simulink model "RaspPiPilot"  (R2014a)
settings: Solver=FixedStepDiscrete  SolverMode=SingleTasking  StartTime=0.0  StopTime=inf  FixedStep=0.2  RelTol=1e-3
PreLoadFcn:
  | load JoystickBus
undefined symbols (not defined in the file or in its folder): fdesignblkfcn, gcbh
libraries: simulink x11, visionstatistics x5, visiontextngfix x2, embdlinuxlib x2
settings Model: SimulationMode=external  ExtModeTrigDuration=100  Creator=jsustare  LastModifiedBy=jsustare
settings OptimizationCC: OptimizeModelRefInitCode=on  LifeSpan=1
settings DebuggingCC: UnderspecifiedInitializationDetection=Classic  SolverPrmCheckMsg=none
settings HardwareCC: ProdLargestAtomicInteger=Long  ProdLargestAtomicFloat=Double  ProdEndianess=LittleEndian  ProdHWDeviceType=ARM Compatible->ARM Cortex
settings RTWCC: SystemTargetFile=realtime.tlc  GenerateMakefile=off  TemplateMakefile=realtime.tmf  Description=Run on Target Hardware  RTWVerbose=off  ProcessScript=realtime_make_rtw_hook  CustomInclude=include include/common  CustomSource=SerialPort.c mavlink.c
settings RTWCC: CustomHeaderCode=|
  | #include <mavlink.h>
  | #include <common.h>
settings STFCustomTargetCC: TargetLibSuffix=.a  GenerateSampleERTMain=on  ConcurrentExecutionCompliant=off  GeneratePreprocessorConditionals=Use local settings  ERTCustomFileBanners=on  SupportNonInlinedSFcns=off  SupportVariableSizeSignals=on  MATLABClassNameForMDSCustomization=Simulink.SoftwareTarget.ERTCustomization  GRTInterface=off  SystemTargetFile=realtime.tlc
settings ERTTargetCC: CombineOutputUpdateFcns=off  SupportContinuousTime=on  SupportVariableSizeSignals=on  ExtMode=on  ExtModeMexArgs='169.254.0.31' 0 17725 30  ERTSrcFileBannerTemplate=realtime_code_template.cgt  ERTHdrFileBannerTemplate=realtime_code_template.cgt  ERTDataSrcFileTemplate=realtime_code_template.cgt  ERTDataHdrFileTemplate=realtime_code_template.cgt  ERTCustomFileTemplate=realtime_file_process.tlc

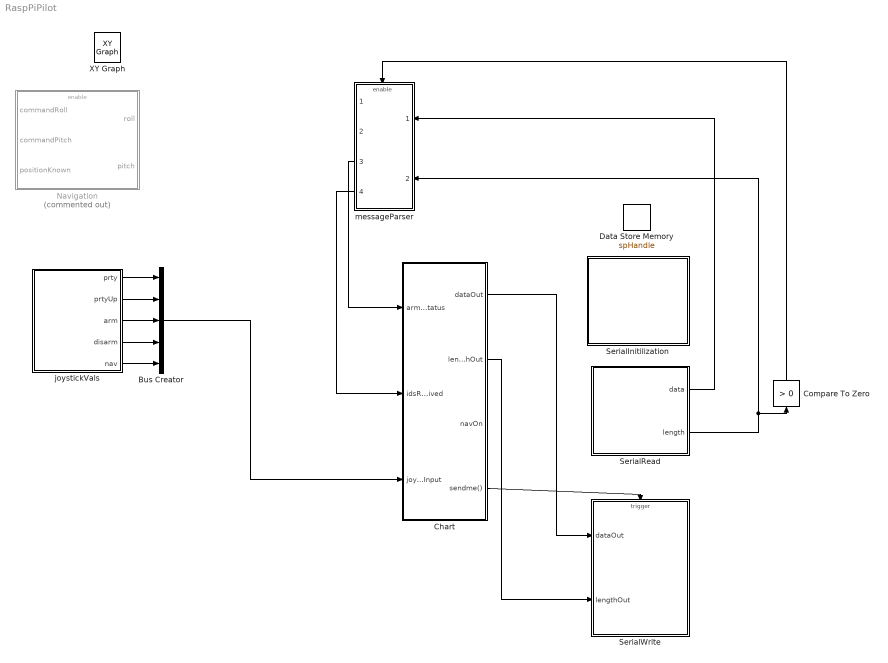
== system RaspPiPilot ==
  Bus Creator : BusCreator  Inputs=5  OutDataTypeStr=Bus: JoystickBus
  Chart : Stateflow chart  TreatAsAtomicUnit=on
  Compare To Zero : simulink/Logic and Bit Operations/Compare To Zero  relop=>  OutDataTypeStr=boolean
  Data Store Memory : DataStoreMemory  DataStoreName=spHandle  ReadBeforeWriteMsg=warning  WriteAfterWriteMsg=warning  WriteAfterReadMsg=warning  InitialValue=-1  OutDataTypeStr=int32
  Navigation : Subsystem  Commented=on
  SerialInitilization : MATLAB Function  TreatAsAtomicUnit=on
  SerialRead : MATLAB Function  TreatAsAtomicUnit=on
  SerialWrite : MATLAB Function  TreatAsAtomicUnit=on
  joystickVals : Subsystem
  messageParser : Subsystem
  XY Graph : simulink/Sinks/XY Graph  IOType=viewer  xmin=-1  xmax=1  ymin=-1  ymax=1  st=-1
  wires:
  Compare To Zero/1 -> messageParser/Enable
  Chart/1(dataOut) -> SerialWrite/1(dataOut)
  Chart/2(lengthOut) -> SerialWrite/2(lengthOut)
  Chart/4(sendme()) -> SerialWrite/Trigger
  SerialRead/2(length) -> messageParser/2(lengthRead), Compare To Zero/1
  SerialRead/1(data) -> messageParser/1("dataRead ")
  messageParser/3(armStatus) -> Chart/1(armStatus)
  messageParser/4(bussyBus) -> Chart/2(idsReceived)
  joystickVals/4(disarm) -> Bus Creator/4
  joystickVals/1(prty) -> Bus Creator/1
  joystickVals/3(arm) -> Bus Creator/3
  joystickVals/2(prtyUp) -> Bus Creator/2
  joystickVals/5(nav) -> Bus Creator/5
  Bus Creator/1 -> Chart/3(joystickInput)

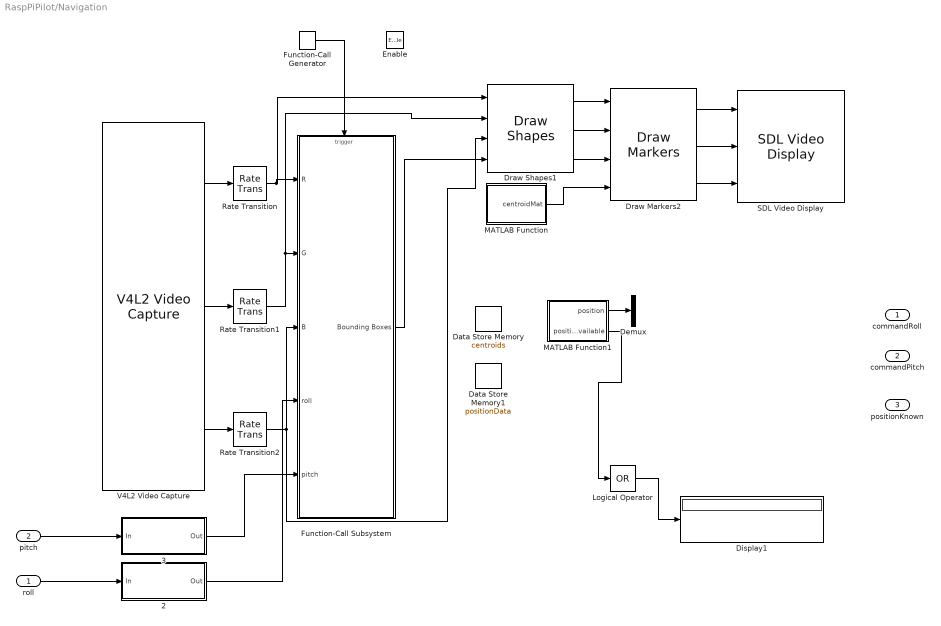
== system RaspPiPilot/Navigation ==
  roll : Inport
  pitch : Inport  Port=2
  Enable : EnablePort  PropagateVarSize=During execution
  " 2" : Subsystem  DialogController=fdesignblkfcn  InitFcn=fdesignblkfcn(gcbh, {'InitFcn'});  mask(Lowpass Filter){}
      mask help: Design a lowpass filter
      settings: CopyFcn=fdesignblkfcn(gcbh, {'CopyFcn'});
      mask Help: helpview(mapfilelocation('dsp'), 'dsplowpassfilter');
      mask Display: disp('Lowpass')
  " 3" : Subsystem  DialogController=fdesignblkfcn  InitFcn=fdesignblkfcn(gcbh, {'InitFcn'});  mask(Lowpass Filter){}
      mask help: Design a lowpass filter
      settings: CopyFcn=fdesignblkfcn(gcbh, {'CopyFcn'});
      mask Help: helpview(mapfilelocation('dsp'), 'dsplowpassfilter');
      mask Display: disp('Lowpass')
  Data Store Memory : DataStoreMemory  DataStoreName=centroids  ReadBeforeWriteMsg=warning  WriteAfterWriteMsg=warning  WriteAfterReadMsg=warning  InitialValue=zeros(13,2,4)  OutDataTypeStr=double
  Data Store Memory1 : DataStoreMemory  DataStoreName=positionData  ReadBeforeWriteMsg=warning  WriteAfterWriteMsg=warning  WriteAfterReadMsg=warning  InitialValue=-1000*ones(4,2)  OutDataTypeStr=double
  Demux : Demux  Outputs=2
  Display1 : Display
  Draw Markers2 : visiontextngfix/Draw Markers  shape=X-mark  size=3  fill=off  fillClrSource=Specify via dialog  display=User-specified value  intensity=200  color=[255 255 255]  opacity=0.6  viewport=Entire image  antialiasing=off  inType=Obsolete  imagePorts=Separate color signals  prodOutputMode=Binary point scaling  prodOutputWordLength=32  prodOutputFracLength=14  memoryMode=Specify word length  memoryWordLength=16  memoryFracLength=15  roundingMode=Floor  overflowMode=off
  Draw Shapes1 : visiontextngfix/Draw Shapes  shape=Rectangles  fill=off  lineWidth=1  fillClrSource=Specify via dialog  display=User-specified value  intensity=200  color=[255 0 0]  opacity=0.6  viewport=Entire image  antialiasing=off  inType=Obsolete  imagePorts=Separate color signals  prodOutputMode=Binary point scaling  prodOutputWordLength=32  prodOutputFracLength=14  memoryMode=Specify word length  memoryWordLength=16  memoryFracLength=15  roundingMode=Floor  overflowMode=off
  Function-Call Generator : simulink/Ports & Subsystems/Function-Call Generator  sample_time=0.2  numberOfIterations=1
  Function-Call Subsystem : Subsystem  TreatAsAtomicUnit=on
  Logical Operator : Logic  Operator=OR  Inputs=1  AllPortsSameDT=off  OutDataTypeStr=boolean
  MATLAB Function : MATLAB Function  TreatAsAtomicUnit=on
  MATLAB Function1 : MATLAB Function  TreatAsAtomicUnit=on
  Rate Transition : RateTransition  Deterministic=off
  Rate Transition1 : RateTransition  Deterministic=off
  Rate Transition2 : RateTransition  Deterministic=off
  SDL Video Display : embdlinuxlib/SDL Video Display  pixelFormat=RGB  pixelOrder=Planar  rowMajor=on  blockPlatform=Raspberry Pi
  V4L2 Video Capture : embdlinuxlib/V4L2 Video Capture  m_devName='/dev/video0'  roi=[0, 0, 640, 480]  imSizeSelection=320x240  imSize=[640, 480]  pixelFormat=RGB  pixelOrder=Planar  sampleTime=0.2  simOutput=Colorbars  blockPlatform=Raspberry Pi
  commandRoll : Outport
  commandPitch : Outport  Port=2
  positionKnown : Outport  Port=3
  wires:
  V4L2 Video Capture/3 -> Rate Transition2/1
  V4L2 Video Capture/1 -> Rate Transition/1
  V4L2 Video Capture/2 -> Rate Transition1/1
  Function-Call Generator/1 -> Function-Call Subsystem/Trigger
  Function-Call Subsystem/1("Bounding Boxes ") -> Draw Shapes1/4
  Rate Transition/1 -> Draw Shapes1/1, Function-Call Subsystem/1(R)
  Rate Transition1/1 -> Draw Shapes1/2, Function-Call Subsystem/2(G)
  Rate Transition2/1 -> Draw Shapes1/3, Function-Call Subsystem/3(B)
  Draw Markers2/2 -> SDL Video Display/2
  Draw Markers2/3 -> SDL Video Display/3
  Draw Markers2/1 -> SDL Video Display/1
  Draw Shapes1/3 -> Draw Markers2/3
  Draw Shapes1/2 -> Draw Markers2/2
  Draw Shapes1/1 -> Draw Markers2/1
  pitch/1 -> " 3"/1(In)
  " 2"/1(Out) -> Function-Call Subsystem/4(roll)
  roll/1 -> " 2"/1(In)
  MATLAB Function/1(centroidMat) -> Draw Markers2/4
  MATLAB Function1/2(positionAvailable) -> Logical Operator/1
  Logical Operator/1 -> Display1/1
  " 3"/1(Out) -> Function-Call Subsystem/5(pitch)
  MATLAB Function1/1(position) -> Demux/1

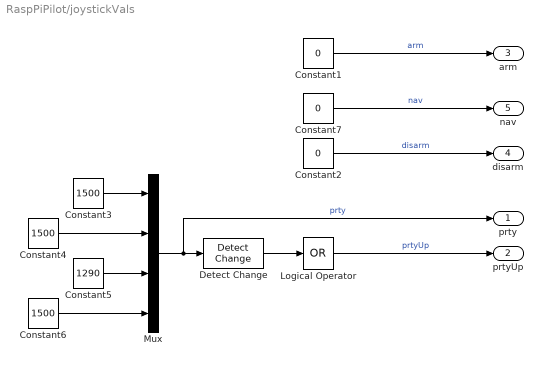
== system RaspPiPilot/joystickVals ==
  Constant1 : Constant  Value=0  OutDataTypeStr=boolean
  Constant2 : Constant  Value=0  OutDataTypeStr=boolean
  Constant3 : Constant  Value=1500
  Constant4 : Constant  Value=1500
  Constant5 : Constant  Value=1290
  Constant6 : Constant  Value=1500
  Constant7 : Constant  Value=0  OutDataTypeStr=boolean
  Detect Change : simulink/Logic and Bit Operations/Detect Change  vinit=0  InputProcessing=Inherited  OutDataTypeStr=boolean
  Logical Operator : Logic  Operator=OR  Inputs=1  AllPortsSameDT=off  OutDataTypeStr=boolean
  Mux : Mux
  prty : Outport
  prtyUp : Outport  Port=2
  arm : Outport  Port=3
  disarm : Outport  Port=4
  nav : Outport  Port=5
  wires:
  Constant3/1 -> Mux/1
  Constant4/1 -> Mux/2
  Constant5/1 -> Mux/3
  Constant6/1 -> Mux/4
  Mux/1 -> prty/1, Detect Change/1  "prty"
  Detect Change/1 -> Logical Operator/1
  Logical Operator/1 -> prtyUp/1  "prtyUp"
  Constant1/1 -> arm/1  "arm"
  Constant2/1 -> disarm/1  "disarm"
  Constant7/1 -> nav/1  "nav"

== system RaspPiPilot/messageParser ==
  "dataRead " : Inport
  lengthRead : Inport  Port=2
  Enable : EnablePort
  While Iterator Subsystem : Subsystem  TreatAsAtomicUnit=on
  rollData : Outport
  pitchData : Outport  Port=2
  armStatus : Outport  Port=3
  bussyBus : Outport  Port=4
  wires:
  "dataRead "/1 -> While Iterator Subsystem/1(DataRead)
  lengthRead/1 -> While Iterator Subsystem/2(lengthRead)
  While Iterator Subsystem/1(roll) -> rollData/1
  While Iterator Subsystem/2(pitch) -> pitchData/1
  While Iterator Subsystem/3(armStatus) -> armStatus/1
  While Iterator Subsystem/4("idsReceived ") -> bussyBus/1

== system RaspPiPilot/Navigation/ 2 ==
  In : Inport
  Generated Filter Block : DiscreteFir  Tag=BlockMethodSubSystem  Coefficients=[0.0032276888738420255 -0.012093185057654832 -0.056871256727662273 -0.033025317279675399 0.16717851315296134 0.40566714821275895 0.40566714821275895 0.16717851315296134 -0.033025317279675399 -0.056871256727662273 -0.012093185057654832 0.0032276888738420255]  InputProcessing=Columns as channels (frame based)
  Out : Outport
  wires:
  Generated Filter Block/1 -> Out/1
  In/1 -> Generated Filter Block/1

== system RaspPiPilot/Navigation/ 3 ==
  In : Inport
  Generated Filter Block : DiscreteFir  Tag=BlockMethodSubSystem  Coefficients=[0.0032276888738420255 -0.012093185057654832 -0.056871256727662273 -0.033025317279675399 0.16717851315296134 0.40566714821275895 0.40566714821275895 0.16717851315296134 -0.033025317279675399 -0.056871256727662273 -0.012093185057654832 0.0032276888738420255]  InputProcessing=Columns as channels (frame based)
  Out : Outport
  wires:
  In/1 -> Generated Filter Block/1
  Generated Filter Block/1 -> Out/1

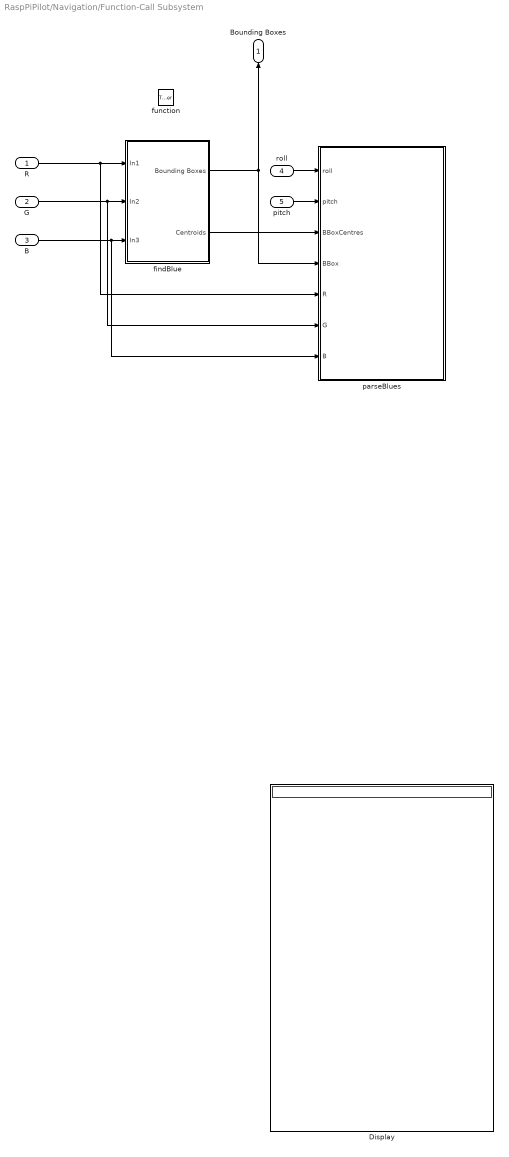
== system RaspPiPilot/Navigation/Function-Call Subsystem ==
  R : Inport
  G : Inport  Port=2
  B : Inport  Port=3
  roll : Inport  Port=4
  pitch : Inport  Port=5
  function : TriggerPort  TriggerType=function-call
  Display : Display
  findBlue : Subsystem
  parseBlues : Subsystem  TreatAsAtomicUnit=on
  "Bounding Boxes " : Outport
  wires:
  G/1 -> parseBlues/6(G), findBlue/2(In2)
  R/1 -> parseBlues/5(R), findBlue/1(In1)
  B/1 -> parseBlues/7(B), findBlue/3(In3)
  findBlue/1(Bounding Boxes) -> parseBlues/4(BBox), "Bounding Boxes "/1
  findBlue/2(Centroids) -> parseBlues/3(BBoxCentres)
  roll/1 -> parseBlues/1(roll)
  pitch/1 -> parseBlues/2(pitch)

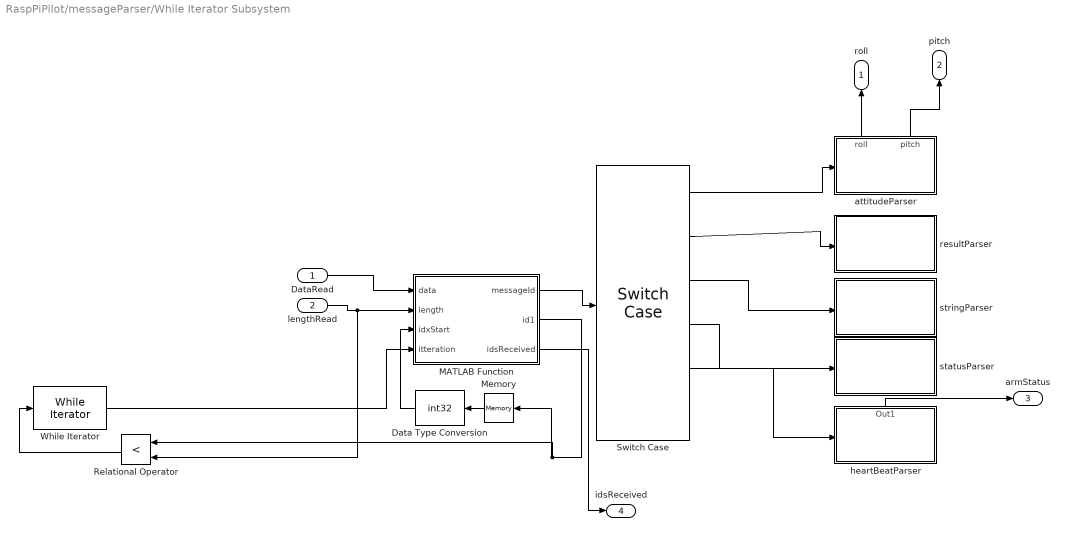
== system RaspPiPilot/messageParser/While Iterator Subsystem ==
  DataRead : Inport
  lengthRead : Inport  Port=2
  Data Type Conversion : DataTypeConversion  OutDataTypeStr=int32
  MATLAB Function : MATLAB Function  TreatAsAtomicUnit=on
  Memory : Memory  X0=1  InheritSampleTime=on
  Relational Operator : RelationalOperator  Operator=<  OutDataTypeStr=boolean
  Switch Case : SwitchCase  CaseConditions={30,77,253,1,0}
  While Iterator : WhileIterator  MaxIters=100  WhileBlockType=do-while  ShowIterationPort=on
  attitudeParser : Subsystem  TreatAsAtomicUnit=on
  heartBeatParser : Subsystem  TreatAsAtomicUnit=on
  resultParser : Subsystem  TreatAsAtomicUnit=on
  statusParser : Subsystem  TreatAsAtomicUnit=on
  stringParser : Subsystem  TreatAsAtomicUnit=on
  roll : Outport
  pitch : Outport  Port=2
  armStatus : Outport  Port=3
  "idsReceived " : Outport  Port=4
  wires:
  DataRead/1 -> MATLAB Function/1(data)
  lengthRead/1 -> Relational Operator/2, MATLAB Function/2(length)
  Relational Operator/1 -> While Iterator/1
  While Iterator/1 -> MATLAB Function/4(itteration)
  Memory/1 -> Data Type Conversion/1
  Data Type Conversion/1 -> MATLAB Function/3(idxStart)
  MATLAB Function/2(id1) -> Relational Operator/1, Memory/1
  MATLAB Function/1(messageId) -> Switch Case/1
  Switch Case/1 -> attitudeParser/Action
  Switch Case/2 -> resultParser/Action
  Switch Case/3 -> stringParser/Action
  Switch Case/4 -> statusParser/Action
  Switch Case/5 -> heartBeatParser/Action
  attitudeParser/1(roll) -> roll/1
  heartBeatParser/1(Out1) -> armStatus/1
  attitudeParser/2(pitch) -> pitch/1
  MATLAB Function/3(idsReceived) -> "idsReceived "/1

== system RaspPiPilot/Navigation/Function-Call Subsystem/findBlue ==
  In1 : Inport
  In2 : Inport  Port=2
  In3 : Inport  Port=3
  Blob Analysis : visionstatistics/Blob Analysis  Tag=vipblks_row_conv  area=on  centroid=on  bBox=on  majorAxis=off  minorAxis=off  angle=off  eccentricity=off  equivDiameterSq=off  extent=off  perimeter=off  maxBlobs=16  warnIfNumBlobsExceeded=on  isCount=off  useMinArea=on  minArea=300  useMaxArea=off  maxArea=intmax('uint32')  excludeBorderBlob=on  outDT=double  isOutVarDim=off  isFill=on  fillValues=-1  conn=8  isLabel=off  outputMode=Binary point scaling  outputWordLength=32  outputFracLength=16  firstCoeffMode=Binary point scaling  firstCoeffWordLength=16  firstCoeffFracLength=14  secondCoeffMode=Binary point scaling  secondCoeffWordLength=32  secondCoeffFracLength=16  accumMode=Binary point scaling  accumWordLength=32  accumFracLength=0  prodOutputMode=Binary point scaling  prodOutputWordLength=32  prodOutputFracLength=16  roundingMode=Floor  overflowMode=off
  Compare To Constant : simulink/Logic and Bit Operations/Compare To Constant  relop=>  const=15  OutDataTypeStr=boolean
  MATLAB Function : MATLAB Function  TreatAsAtomicUnit=on
  MATLAB Function1 : MATLAB Function  TreatAsAtomicUnit=on
  Bounding Boxes : Outport
  Centroids : Outport  Port=2
  wires:
  Compare To Constant/1 -> Blob Analysis/1
  Blob Analysis/3 -> MATLAB Function/3(bbox)
  Blob Analysis/1 -> MATLAB Function/1(area)
  MATLAB Function/2(bbox_largest) -> Bounding Boxes/1
  MATLAB Function/1(centroid_largest) -> Centroids/1
  Blob Analysis/2 -> MATLAB Function/2(centroid)
  MATLAB Function1/1(blueIntensity) -> Compare To Constant/1
  In1/1 -> MATLAB Function1/1(R)
  In2/1 -> MATLAB Function1/2(G)
  In3/1 -> MATLAB Function1/3(B)

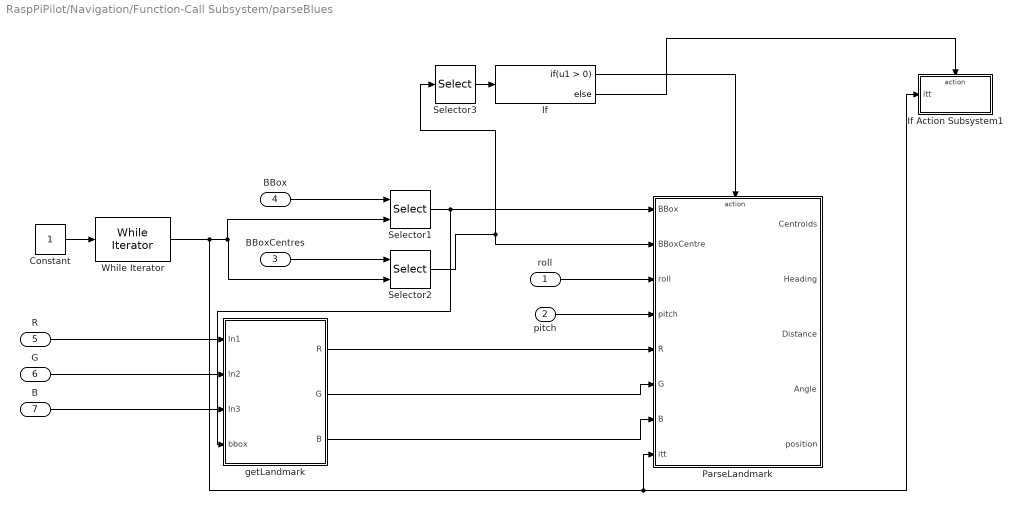
== system RaspPiPilot/Navigation/Function-Call Subsystem/parseBlues ==
  roll : Inport
  pitch : Inport  Port=2
  BBoxCentres : Inport  Port=3
  BBox : Inport  Port=4
  R : Inport  Port=5
  G : Inport  Port=6
  B : Inport  Port=7
  Constant : Constant
  If : If
  If Action Subsystem1 : Subsystem  TreatAsAtomicUnit=on
  ParseLandmark : Subsystem  TreatAsAtomicUnit=on
  Selector1 : Selector  NumberOfDimensions=2  InputPortWidth=3  IndexOptions=Index vector (port),Select all  Indices=[1 3],1  OutputSizes=1,1
  Selector2 : Selector  NumberOfDimensions=2  InputPortWidth=3  IndexOptions=Index vector (port),Select all  Indices=[1 3],1  OutputSizes=1,1
  Selector3 : Selector  InputPortWidth=2
  While Iterator : WhileIterator  MaxIters=4  WhileBlockType=do-while  ShowIterationPort=on
  getLandmark : Subsystem
  wires:
  roll/1 -> ParseLandmark/3(roll)
  pitch/1 -> ParseLandmark/4(pitch)
  While Iterator/1 -> ParseLandmark/8("itt "), If Action Subsystem1/1(itt), Selector1/2, Selector2/2
  BBox/1 -> Selector1/1
  BBoxCentres/1 -> Selector2/1
  Selector1/1 -> ParseLandmark/1(BBox), getLandmark/4(bbox)
  Selector2/1 -> Selector3/1, ParseLandmark/2(BBoxCentre)
  R/1 -> getLandmark/1(In1)
  G/1 -> getLandmark/2(In2)
  B/1 -> getLandmark/3(In3)
  Constant/1 -> While Iterator/1
  getLandmark/1(R) -> ParseLandmark/5(R)
  getLandmark/2(G) -> ParseLandmark/6(G)
  getLandmark/3(B) -> ParseLandmark/7(B)
  If/1 -> ParseLandmark/Action
  If/2 -> If Action Subsystem1/Action
  Selector3/1 -> If/1

== system RaspPiPilot/messageParser/While Iterator Subsystem/attitudeParser ==
  Action Port : ActionPort  ActionType=case
  MATLAB Function1 : MATLAB Function  TreatAsAtomicUnit=on
  roll : Outport
  pitch : Outport  Port=2
  wires:
  MATLAB Function1/1(roll) -> roll/1
  MATLAB Function1/2(pitch) -> pitch/1

== system RaspPiPilot/messageParser/While Iterator Subsystem/heartBeatParser ==
  Action Port : ActionPort  ActionType=case
  MATLAB Function1 : MATLAB Function  TreatAsAtomicUnit=on
  Out1 : Outport
  wires:
  MATLAB Function1/1(armed) -> Out1/1

== system RaspPiPilot/messageParser/While Iterator Subsystem/resultParser ==
  Action Port : ActionPort  ActionType=case
  MATLAB Function1 : MATLAB Function  TreatAsAtomicUnit=on

== system RaspPiPilot/messageParser/While Iterator Subsystem/statusParser ==
  Action Port : ActionPort  ActionType=case
  MATLAB Function1 : MATLAB Function  TreatAsAtomicUnit=on

== system RaspPiPilot/messageParser/While Iterator Subsystem/stringParser ==
  Action Port : ActionPort  ActionType=case
  MATLAB Function1 : MATLAB Function  TreatAsAtomicUnit=on

== system RaspPiPilot/Navigation/Function-Call Subsystem/parseBlues/If Action Subsystem1 ==
  itt : Inport
  Action Port : ActionPort  ActionType=else
  MATLAB Function1 : MATLAB Function  TreatAsAtomicUnit=on
  wires:
  itt/1 -> MATLAB Function1/1(itt)

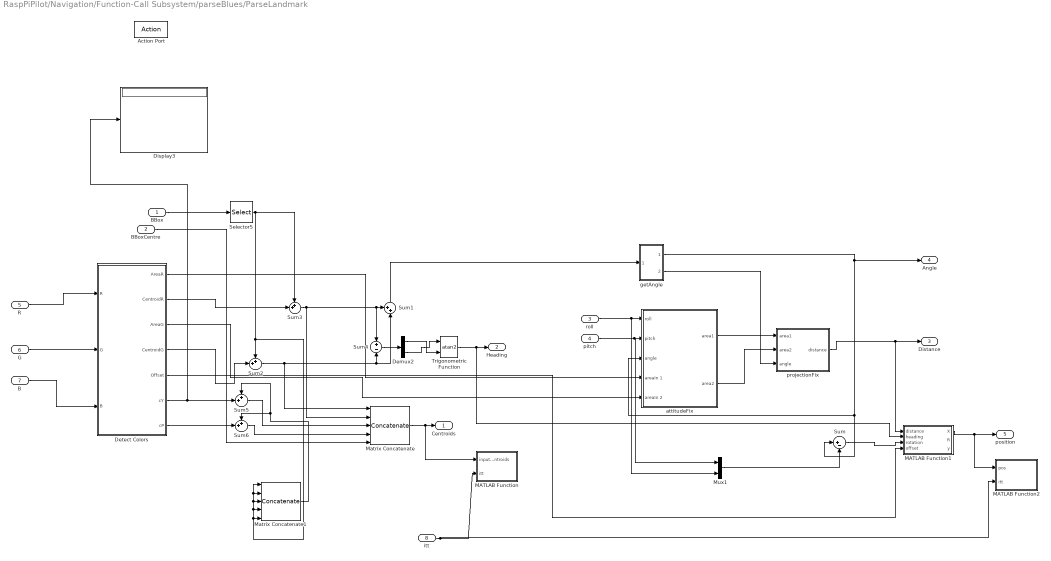
== system RaspPiPilot/Navigation/Function-Call Subsystem/parseBlues/ParseLandmark ==
  BBox : Inport
  BBoxCentre : Inport  Port=2
  roll : Inport  Port=3
  pitch : Inport  Port=4
  R : Inport  Port=5
  G : Inport  Port=6
  B : Inport  Port=7
  "itt " : Inport  Port=8
  Action Port : ActionPort  PropagateVarSize=During execution  ActionType=then
  Demux2 : Demux  Outputs=2
  Detect Colors : Subsystem
  Display3 : Display
  MATLAB Function : MATLAB Function  TreatAsAtomicUnit=on
  MATLAB Function1 : MATLAB Function  TreatAsAtomicUnit=on
  MATLAB Function2 : MATLAB Function  TreatAsAtomicUnit=on
  Matrix Concatenate : Concatenate  NumInputs=5  Mode=Multidimensional array
  Matrix Concatenate1 : Concatenate  NumInputs=5  Mode=Multidimensional array
  Mux1 : Mux  Inputs=2
  Selector5 : Selector  InputPortWidth=4  Indices=[1 2]
  Sum : Sum  Inputs=|+-
  Sum{1..3,5..6} (5 alike) : Sum  Inputs=++|
  Sum4 : Sum  Inputs=+-
  Trigonometric Function : Trigonometry  Operator=atan2
  attitudeFix : Subsystem
  getAngle : Subsystem
  projectionFix : Subsystem
  Centroids : Outport
  Heading : Outport  Port=2
  "Distance " : Outport  Port=3
  Angle : Outport  Port=4
  position : Outport  Port=5
  wires:
  Detect Colors/5(Offset) -> MATLAB Function1/4(offset)
  B/1 -> Detect Colors/3(B)
  G/1 -> Detect Colors/2(G)
  R/1 -> Detect Colors/1(R)
  Matrix Concatenate1/1 -> Sum5/1, Sum6/1
  Selector5/1 -> Sum2/1, Matrix Concatenate1/1, Matrix Concatenate1/2, Matrix Concatenate1/3, Matrix Concatenate1/4, Matrix Concatenate1/5, Sum3/1
  BBoxCentre/1 -> Matrix Concatenate/5
  Sum5/1 -> Matrix Concatenate/3
  Sum6/1 -> Matrix Concatenate/4
  Detect Colors/7(cP) -> Sum6/2
  Detect Colors/6(cY) -> Sum5/2, Display3/1
  MATLAB Function1/1(X) -> MATLAB Function2/1(pos), position/1
  Trigonometric Function/1 -> Heading/1, MATLAB Function1/2(heading)
  roll/1 -> attitudeFix/1(roll), Mux1/2
  Mux1/1 -> Sum/2
  Sum/1 -> MATLAB Function1/3(rotation)
  Detect Colors/3(AreaG) -> attitudeFix/5(areaIn 2)
  Sum2/1 -> Sum4/2, Sum1/2, Matrix Concatenate/1
  Detect Colors/4(CentroidG) -> Sum2/2
  BBox/1 -> Selector5/1
  projectionFix/1(distance) -> "Distance "/1, MATLAB Function1/1(distance)
  Detect Colors/1(AreaR) -> attitudeFix/4(areaIn 1)
  Sum3/1 -> Sum4/1, Sum1/1, Matrix Concatenate/2
  Detect Colors/2(CentroidR) -> Sum3/2
  Demux2/1 -> Trigonometric Function/2
  Demux2/2 -> Trigonometric Function/1
  Sum4/1 -> Demux2/1
  attitudeFix/2(area2) -> projectionFix/2(area2)
  attitudeFix/1(area1) -> projectionFix/1(area1)
  pitch/1 -> attitudeFix/2(pitch), Mux1/1
  Matrix Concatenate/1 -> MATLAB Function/1(inputCentroids), Centroids/1
  "itt "/1 -> MATLAB Function2/2(itt), MATLAB Function/2(itt)
  getAngle/1(Out1) -> attitudeFix/3("angle "), Sum/1, Angle/1
  Sum1/1 -> getAngle/1(In1)
  getAngle/2(Out2) -> projectionFix/3(angle)

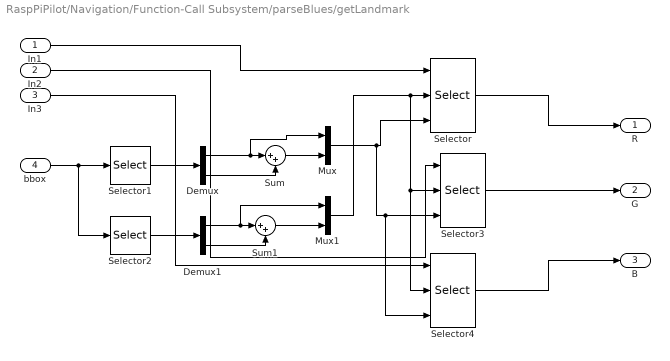
== system RaspPiPilot/Navigation/Function-Call Subsystem/parseBlues/getLandmark ==
  In1 : Inport
  In2 : Inport  Port=2
  In3 : Inport  Port=3
  bbox : Inport  Port=4
  Demux : Demux  Outputs=2
  Demux1 : Demux  Outputs=2
  Mux : Mux  Inputs=2
  Mux1 : Mux  Inputs=2
  Selector : Selector  NumberOfDimensions=2  InputPortWidth=3  IndexOptions=Starting and ending indices (port),Starting and ending indices (port)  Indices=[1 3],1  OutputSizes=1,1
  Selector1 : Selector  InputPortWidth=4  Indices=[1 3]
  Selector2 : Selector  InputPortWidth=4  Indices=[2 4]
  Selector3 : Selector  NumberOfDimensions=2  InputPortWidth=3  IndexOptions=Starting and ending indices (port),Starting and ending indices (port)  Indices=[1 3],1  OutputSizes=1,1
  Selector4 : Selector  NumberOfDimensions=2  InputPortWidth=3  IndexOptions=Starting and ending indices (port),Starting and ending indices (port)  Indices=[1 3],1  OutputSizes=1,1
  Sum : Sum  Inputs=|++
  Sum1 : Sum  Inputs=|++
  R : Outport
  G : Outport  Port=2
  B : Outport  Port=3
  wires:
  In1/1 -> Selector/1
  In2/1 -> Selector3/1
  In3/1 -> Selector4/1
  bbox/1 -> Selector2/1, Selector1/1
  Selector1/1 -> Demux/1
  Selector2/1 -> Demux1/1
  Demux/1 -> Mux/1, Sum/1
  Demux/2 -> Sum/2
  Demux1/1 -> Mux1/1, Sum1/1
  Demux1/2 -> Sum1/2
  Sum/1 -> Mux/2
  Sum1/1 -> Mux1/2
  Selector/1 -> R/1
  Selector3/1 -> G/1
  Selector4/1 -> B/1
  Mux/1 -> Selector4/3, Selector3/3, Selector/3
  Mux1/1 -> Selector4/2, Selector3/2, Selector/2

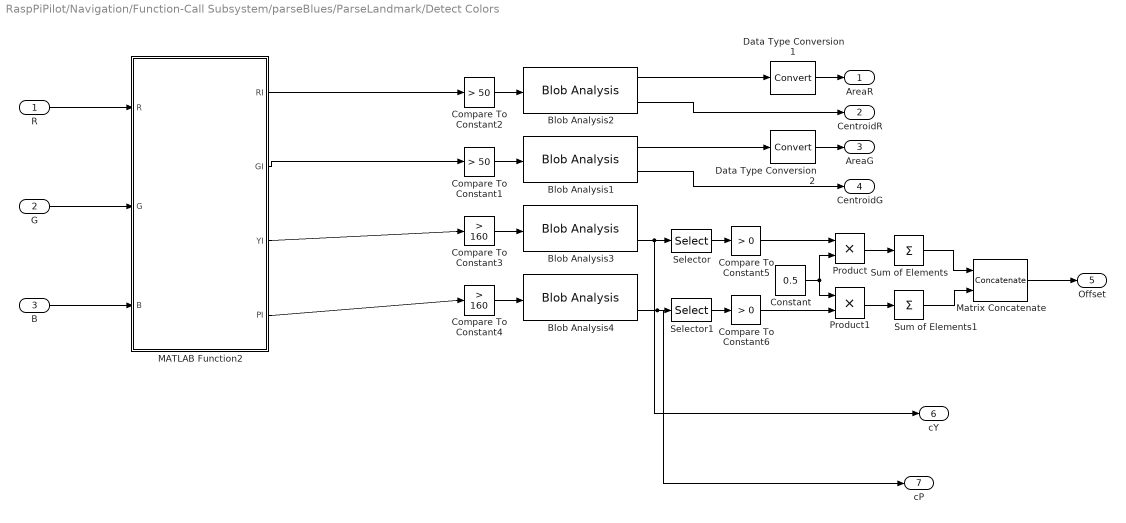
== system RaspPiPilot/Navigation/Function-Call Subsystem/parseBlues/ParseLandmark/Detect Colors ==
  R : Inport
  G : Inport  Port=2
  B : Inport  Port=3
  Blob Analysis1 : visionstatistics/Blob Analysis  Tag=vipblks_row_conv  area=on  centroid=on  bBox=off  majorAxis=off  minorAxis=off  angle=off  eccentricity=off  equivDiameterSq=off  extent=off  perimeter=off  maxBlobs=1  warnIfNumBlobsExceeded=on  isCount=off  useMinArea=off  minArea=0  useMaxArea=off  maxArea=intmax('uint32')  excludeBorderBlob=off  outDT=double  isOutVarDim=off  isFill=on  fillValues=-1  conn=8  isLabel=off  outputMode=Binary point scaling  outputWordLength=32  outputFracLength=16  firstCoeffMode=Binary point scaling  firstCoeffWordLength=16  firstCoeffFracLength=14  secondCoeffMode=Binary point scaling  secondCoeffWordLength=32  secondCoeffFracLength=16  accumMode=Binary point scaling  accumWordLength=32  accumFracLength=0  prodOutputMode=Binary point scaling  prodOutputWordLength=32  prodOutputFracLength=16  roundingMode=Floor  overflowMode=off
  Blob Analysis2 : visionstatistics/Blob Analysis  Tag=vipblks_row_conv  area=on  centroid=on  bBox=off  majorAxis=off  minorAxis=off  angle=off  eccentricity=off  equivDiameterSq=off  extent=off  perimeter=off  maxBlobs=1  warnIfNumBlobsExceeded=on  isCount=off  useMinArea=off  minArea=0  useMaxArea=off  maxArea=intmax('uint32')  excludeBorderBlob=off  outDT=double  isOutVarDim=off  isFill=on  fillValues=-1  conn=8  isLabel=off  outputMode=Binary point scaling  outputWordLength=32  outputFracLength=16  firstCoeffMode=Binary point scaling  firstCoeffWordLength=16  firstCoeffFracLength=14  secondCoeffMode=Binary point scaling  secondCoeffWordLength=32  secondCoeffFracLength=16  accumMode=Binary point scaling  accumWordLength=32  accumFracLength=0  prodOutputMode=Binary point scaling  prodOutputWordLength=32  prodOutputFracLength=16  roundingMode=Floor  overflowMode=off
  Blob Analysis3 : visionstatistics/Blob Analysis  Tag=vipblks_row_conv  area=on  centroid=on  bBox=off  majorAxis=off  minorAxis=off  angle=off  eccentricity=off  equivDiameterSq=off  extent=off  perimeter=off  maxBlobs=5  warnIfNumBlobsExceeded=on  isCount=off  useMinArea=on  minArea=10  useMaxArea=off  maxArea=intmax('uint32')  excludeBorderBlob=off  outDT=double  isOutVarDim=off  isFill=on  fillValues=-1  conn=8  isLabel=off  outputMode=Binary point scaling  outputWordLength=32  outputFracLength=16  firstCoeffMode=Binary point scaling  firstCoeffWordLength=16  firstCoeffFracLength=14  secondCoeffMode=Binary point scaling  secondCoeffWordLength=32  secondCoeffFracLength=16  accumMode=Binary point scaling  accumWordLength=32  accumFracLength=0  prodOutputMode=Binary point scaling  prodOutputWordLength=32  prodOutputFracLength=16  roundingMode=Floor  overflowMode=off
  Blob Analysis4 : visionstatistics/Blob Analysis  Tag=vipblks_row_conv  area=on  centroid=on  bBox=off  majorAxis=off  minorAxis=off  angle=off  eccentricity=off  equivDiameterSq=off  extent=off  perimeter=off  maxBlobs=5  warnIfNumBlobsExceeded=on  isCount=off  useMinArea=on  minArea=10  useMaxArea=off  maxArea=intmax('uint32')  excludeBorderBlob=off  outDT=double  isOutVarDim=off  isFill=on  fillValues=-1  conn=8  isLabel=off  outputMode=Binary point scaling  outputWordLength=32  outputFracLength=16  firstCoeffMode=Binary point scaling  firstCoeffWordLength=16  firstCoeffFracLength=14  secondCoeffMode=Binary point scaling  secondCoeffWordLength=32  secondCoeffFracLength=16  accumMode=Binary point scaling  accumWordLength=32  accumFracLength=0  prodOutputMode=Binary point scaling  prodOutputWordLength=32  prodOutputFracLength=16  roundingMode=Floor  overflowMode=off
  Compare To Constant1 : simulink/Logic and Bit Operations/Compare To Constant  relop=>  const=50  OutDataTypeStr=boolean
  Compare To Constant2 : simulink/Logic and Bit Operations/Compare To Constant  relop=>  const=50  OutDataTypeStr=boolean
  Compare To Constant3 : simulink/Logic and Bit Operations/Compare To Constant  relop=>  const=160  OutDataTypeStr=boolean
  Compare To Constant4 : simulink/Logic and Bit Operations/Compare To Constant  relop=>  const=160  OutDataTypeStr=boolean
  Compare To Constant5 : simulink/Logic and Bit Operations/Compare To Constant  relop=>  const=0  OutDataTypeStr=boolean
  Compare To Constant6 : simulink/Logic and Bit Operations/Compare To Constant  relop=>  const=0  OutDataTypeStr=boolean
  Constant : Constant  Value=0.5
  Data Type Conversion1 : DataTypeConversion
  Data Type Conversion2 : DataTypeConversion
  MATLAB Function2 : MATLAB Function  TreatAsAtomicUnit=on
  Matrix Concatenate : Concatenate  Mode=Multidimensional array  ConcatenateDimension=2
  Product : Product
  Product1 : Product
  Selector : Selector  NumberOfDimensions=2  InputPortWidth=3  IndexOptions=Select all,Index vector (dialog)  Indices=1,1  OutputSizes=1,1
  Selector1 : Selector  NumberOfDimensions=2  InputPortWidth=3  IndexOptions=Select all,Index vector (dialog)  Indices=1,1  OutputSizes=1,1
  Sum of Elements : Sum  Inputs=+
  Sum of Elements1 : Sum  Inputs=+
  AreaR : Outport
  CentroidR : Outport  Port=2
  AreaG : Outport  Port=3
  CentroidG : Outport  Port=4
  Offset : Outport  Port=5
  cY : Outport  Port=6
  cP : Outport  Port=7
  wires:
  B/1 -> MATLAB Function2/3(B)
  G/1 -> MATLAB Function2/2(G)
  R/1 -> MATLAB Function2/1(R)
  Matrix Concatenate/1 -> Offset/1
  Sum of Elements1/1 -> Matrix Concatenate/2
  Sum of Elements/1 -> Matrix Concatenate/1
  Product1/1 -> Sum of Elements1/1
  Product/1 -> Sum of Elements/1
  Constant/1 -> Product/2, Product1/1
  Compare To Constant6/1 -> Product1/2
  Compare To Constant5/1 -> Product/1
  Selector1/1 -> Compare To Constant6/1
  Selector/1 -> Compare To Constant5/1
  Blob Analysis4/2 -> Selector1/1, cP/1
  Blob Analysis3/2 -> Selector/1, cY/1
  MATLAB Function2/4(PI) -> Compare To Constant4/1
  Compare To Constant4/1 -> Blob Analysis4/1
  MATLAB Function2/3(YI) -> Compare To Constant3/1
  Compare To Constant3/1 -> Blob Analysis3/1
  MATLAB Function2/2(GI) -> Compare To Constant1/1
  Data Type Conversion2/1 -> AreaG/1
  Blob Analysis1/1 -> Data Type Conversion2/1
  Blob Analysis1/2 -> CentroidG/1
  Compare To Constant1/1 -> Blob Analysis1/1
  Data Type Conversion1/1 -> AreaR/1
  Blob Analysis2/1 -> Data Type Conversion1/1
  Blob Analysis2/2 -> CentroidR/1
  Compare To Constant2/1 -> Blob Analysis2/1
  MATLAB Function2/1(RI) -> Compare To Constant2/1

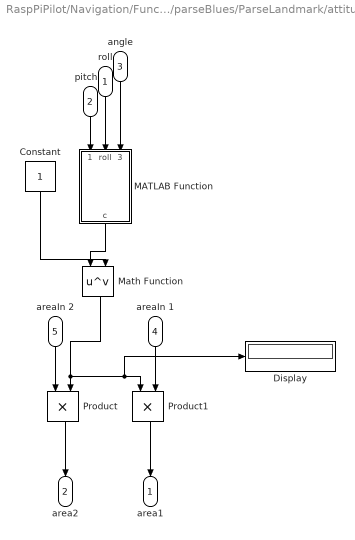
== system RaspPiPilot/Navigation/Function-Call Subsystem/parseBlues/ParseLandmark/attitudeFix ==
  roll : Inport
  pitch : Inport  Port=2
  "angle " : Inport  Port=3
  areaIn 1 : Inport  Port=4
  areaIn 2 : Inport  Port=5
  Constant : Constant
  Display : Display
  MATLAB Function : MATLAB Function  TreatAsAtomicUnit=on
  Math Function : Math  Operator=pow  SaturateOnIntegerOverflow=on
  Product : Product
  Product1 : Product
  area1 : Outport
  area2 : Outport  Port=2
  wires:
  Math Function/1 -> Product/2, Product1/1, Display/1
  Constant/1 -> Math Function/2
  MATLAB Function/1(c) -> Math Function/1
  areaIn 1/1 -> Product1/2
  areaIn 2/1 -> Product/1
  Product/1 -> area2/1
  Product1/1 -> area1/1
  "angle "/1 -> MATLAB Function/3(angle)
  roll/1 -> MATLAB Function/2(roll)
  pitch/1 -> MATLAB Function/1(pitch)

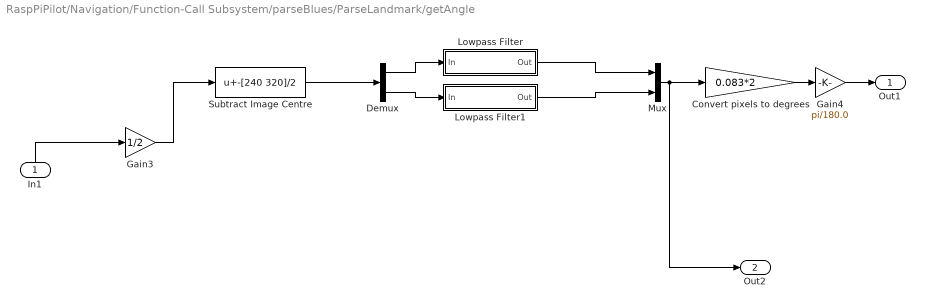
== system RaspPiPilot/Navigation/Function-Call Subsystem/parseBlues/ParseLandmark/getAngle ==
  In1 : Inport
  Convert pixels to degrees : Gain  Gain=0.083*2
  Demux : Demux  Outputs=2
  Gain3 : Gain  Gain=1/2
  Gain4 : Gain  Gain=pi/180.0
  Lowpass Filter : Subsystem  DialogController=fdesignblkfcn  InitFcn=fdesignblkfcn(gcbh, {'InitFcn'});  mask(Lowpass Filter){}
      mask help: Design a lowpass filter
      settings: CopyFcn=fdesignblkfcn(gcbh, {'CopyFcn'});
      mask Help: helpview(mapfilelocation('dsp'), 'dsplowpassfilter');
      mask Display: disp('Lowpass')
  Lowpass Filter1 : Subsystem  DialogController=fdesignblkfcn  InitFcn=fdesignblkfcn(gcbh, {'InitFcn'});  mask(Lowpass Filter){}
      mask help: Design a lowpass filter
      settings: CopyFcn=fdesignblkfcn(gcbh, {'CopyFcn'});
      mask Help: helpview(mapfilelocation('dsp'), 'dsplowpassfilter');
      mask Display: disp('Lowpass')
  Mux : Mux  Inputs=2
  Subtract Image Centre : Bias  Bias=-[240 320]/2
  Out1 : Outport
  Out2 : Outport  Port=2
  wires:
  Gain4/1 -> Out1/1
  Convert pixels to degrees/1 -> Gain4/1
  Subtract Image Centre/1 -> Demux/1
  Gain3/1 -> Subtract Image Centre/1
  In1/1 -> Gain3/1
  Lowpass Filter1/1(Out) -> Mux/2
  Lowpass Filter/1(Out) -> Mux/1
  Demux/1 -> Lowpass Filter/1(In)
  Demux/2 -> Lowpass Filter1/1(In)
  Mux/1 -> Out2/1, Convert pixels to degrees/1

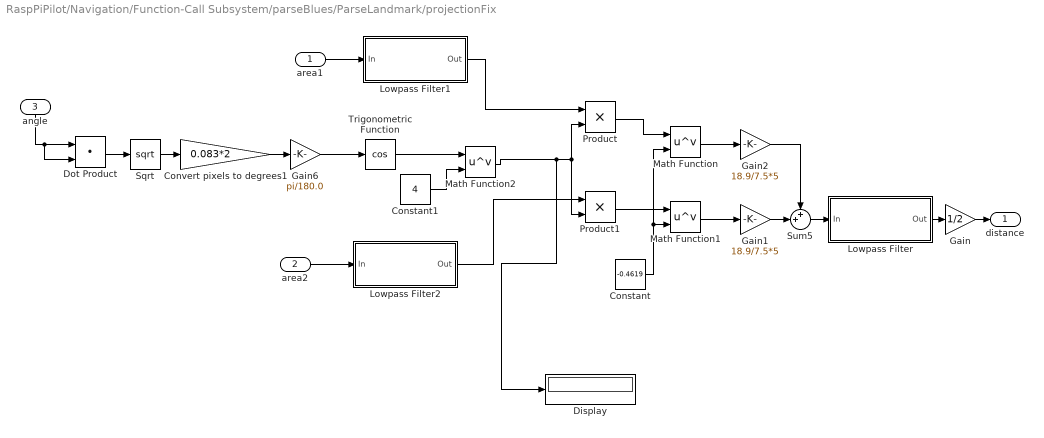
== system RaspPiPilot/Navigation/Function-Call Subsystem/parseBlues/ParseLandmark/projectionFix ==
  area1 : Inport
  area2 : Inport  Port=2
  angle : Inport  Port=3
  Constant : Constant  Value=-0.4619
  Constant1 : Constant  Value=4
  Convert pixels to degrees1 : Gain  Gain=0.083*2
  Display : Display
  Dot Product : DotProduct  InputSameDT=on  OutDataTypeStr=Inherit: Inherit via internal rule
  Gain : Gain  Gain=1/2
  Gain1 : Gain  Gain=18.9/7.5*5
  Gain2 : Gain  Gain=18.9/7.5*5
  Gain6 : Gain  Gain=pi/180.0
  Lowpass Filter : Subsystem  DialogController=fdesignblkfcn  InitFcn=fdesignblkfcn(gcbh, {'InitFcn'});  mask(Lowpass Filter){}
      mask help: Design a lowpass filter
      settings: CopyFcn=fdesignblkfcn(gcbh, {'CopyFcn'});
      mask Help: helpview(mapfilelocation('dsp'), 'dsplowpassfilter');
      mask Display: disp('Lowpass')
  Lowpass Filter1 : Subsystem  DialogController=fdesignblkfcn  InitFcn=fdesignblkfcn(gcbh, {'InitFcn'});  mask(Lowpass Filter){}
      mask help: Design a lowpass filter
      settings: CopyFcn=fdesignblkfcn(gcbh, {'CopyFcn'});
      mask Help: helpview(mapfilelocation('dsp'), 'dsplowpassfilter');
      mask Display: disp('Lowpass')
  Lowpass Filter2 : Subsystem  DialogController=fdesignblkfcn  InitFcn=fdesignblkfcn(gcbh, {'InitFcn'});  mask(Lowpass Filter){}
      mask help: Design a lowpass filter
      settings: CopyFcn=fdesignblkfcn(gcbh, {'CopyFcn'});
      mask Help: helpview(mapfilelocation('dsp'), 'dsplowpassfilter');
      mask Display: disp('Lowpass')
  Math Function : Math  Operator=pow  SaturateOnIntegerOverflow=on
  Math Function1 : Math  Operator=pow  SaturateOnIntegerOverflow=on
  Math Function2 : Math  Operator=pow  SaturateOnIntegerOverflow=on
  Product : Product
  Product1 : Product
  Sqrt : Sqrt  SaturateOnIntegerOverflow=on
  Sum5 : Sum  Inputs=++|
  Trigonometric Function : Trigonometry  Operator=cos
  distance : Outport
  wires:
  Constant1/1 -> Math Function2/2
  Lowpass Filter2/1(Out) -> Product1/1
  Lowpass Filter1/1(Out) -> Product/1
  Trigonometric Function/1 -> Math Function2/1
  Math Function2/1 -> Product1/2, Product/2, Display/1
  Product1/1 -> Math Function1/1
  Product/1 -> Math Function/1
  Sum5/1 -> Lowpass Filter/1(In)
  Sqrt/1 -> Convert pixels to degrees1/1
  Dot Product/1 -> Sqrt/1
  Gain6/1 -> Trigonometric Function/1
  Convert pixels to degrees1/1 -> Gain6/1
  Lowpass Filter/1(Out) -> Gain/1
  Gain1/1 -> Sum5/2
  Gain2/1 -> Sum5/1
  Gain/1 -> distance/1
  area2/1 -> Lowpass Filter2/1(In)
  area1/1 -> Lowpass Filter1/1(In)
  Constant/1 -> Math Function1/2, Math Function/2
  Math Function/1 -> Gain2/1
  Math Function1/1 -> Gain1/1
  angle/1 -> Dot Product/1, Dot Product/2

== system RaspPiPilot/Navigation/Function-Call Subsystem/parseBlues/ParseLandmark/getAngle/Lowpass Filter ==
  In : Inport
  Generated Filter Block : DiscreteFir  Tag=BlockMethodSubSystem  Coefficients=[0.0032276888738420255 -0.012093185057654832 -0.056871256727662273 -0.033025317279675399 0.16717851315296134 0.40566714821275895 0.40566714821275895 0.16717851315296134 -0.033025317279675399 -0.056871256727662273 -0.012093185057654832 0.0032276888738420255]  InputProcessing=Columns as channels (frame based)
  Out : Outport
  wires:
  Generated Filter Block/1 -> Out/1
  In/1 -> Generated Filter Block/1

== system RaspPiPilot/Navigation/Function-Call Subsystem/parseBlues/ParseLandmark/getAngle/Lowpass Filter1 ==
  In : Inport
  Generated Filter Block : DiscreteFir  Tag=BlockMethodSubSystem  Coefficients=[0.0032276888738420255 -0.012093185057654832 -0.056871256727662273 -0.033025317279675399 0.16717851315296134 0.40566714821275895 0.40566714821275895 0.16717851315296134 -0.033025317279675399 -0.056871256727662273 -0.012093185057654832 0.0032276888738420255]  InputProcessing=Columns as channels (frame based)
  Out : Outport
  wires:
  In/1 -> Generated Filter Block/1
  Generated Filter Block/1 -> Out/1

== system RaspPiPilot/Navigation/Function-Call Subsystem/parseBlues/ParseLandmark/projectionFix/Lowpass Filter ==
  In : Inport
  Generated Filter Block : DiscreteFir  Tag=BlockMethodSubSystem  Coefficients=[0.011901508381575016 0.02908797826733928 0.0025913585662860131 -0.068996275507793012 -0.050025679925086837 0.16540100530640869 0.41332778671981452 0.41332778671981452 0.16540100530640869 -0.050025679925086837 -0.068996275507793012 0.0025913585662860131 0.02908797826733928 0.011901508381575016]  InputProcessing=Columns as channels (frame based)
  Out : Outport
  wires:
  Generated Filter Block/1 -> Out/1
  In/1 -> Generated Filter Block/1

== system RaspPiPilot/Navigation/Function-Call Subsystem/parseBlues/ParseLandmark/projectionFix/Lowpass Filter1 ==
  In : Inport
  Generated Filter Block : DiscreteFir  Tag=BlockMethodSubSystem  Coefficients=[0.011901508381575016 0.02908797826733928 0.0025913585662860131 -0.068996275507793012 -0.050025679925086837 0.16540100530640869 0.41332778671981452 0.41332778671981452 0.16540100530640869 -0.050025679925086837 -0.068996275507793012 0.0025913585662860131 0.02908797826733928 0.011901508381575016]  InputProcessing=Columns as channels (frame based)
  Out : Outport
  wires:
  In/1 -> Generated Filter Block/1
  Generated Filter Block/1 -> Out/1

== system RaspPiPilot/Navigation/Function-Call Subsystem/parseBlues/ParseLandmark/projectionFix/Lowpass Filter2 ==
  In : Inport
  Generated Filter Block : DiscreteFir  Tag=BlockMethodSubSystem  Coefficients=[0.011901508381575016 0.02908797826733928 0.0025913585662860131 -0.068996275507793012 -0.050025679925086837 0.16540100530640869 0.41332778671981452 0.41332778671981452 0.16540100530640869 -0.050025679925086837 -0.068996275507793012 0.0025913585662860131 0.02908797826733928 0.011901508381575016]  InputProcessing=Columns as channels (frame based)
  Out : Outport
  wires:
  Generated Filter Block/1 -> Out/1
  In/1 -> Generated Filter Block/1

== matlab function RaspPiPilot/messageParser/While Iterator Subsystem/MATLAB Function ==
  data: data input; messageId output; length input; idxStart input; id1 output; itteration input; idsReceived output size=256
function [messageId,id1,idsReceived]  = parseMavlink(data, length, idxStart,itteration)
messageId=uint8(21);
id1=int32(1);
persistent ids;
if isempty(ids)
    ids=zeros(256,1,'uint8');
end
if itteration==1
    idxStart=itteration;
    ids=zeros(256,1,'uint8');
    
end
if ~coder.target('SFun')
    for i=idxStart:length
        tempD=uint8(0);
        tempD=coder.ceval('parseMavlink',data(i));         
        if tempD>0
            messageId = coder.ceval('getMessageId',i,length);
            ids(messageId+1)=uint8(1);
            if i==length
                id1=i;
            else
                id1=i+1;
            end            
            break;
        else
            id1=i;% if itteration finishes without id trigger - 
        end         
    end     
end
idsReceived=ids;

== matlab function RaspPiPilot/SerialWrite ==
  data: dataOut input; lengthOut input; spHandle data_store_memory
  events: trigger input FUNCTION_CALL_EVENT
function serialWrite(dataOut, lengthOut)
global spHandle;
if ~coder.target('SFun')  
        if lengthOut>0           
            data2=uint8(dataOut);
            coder.ceval('write',spHandle, coder.ref(data2), uint32(lengthOut));
            coder.ceval('debugg');
        end   
end

== matlab function RaspPiPilot/messageParser/While Iterator Subsystem/resultParser/MATLAB Function1 ==
  data: result output
function result  = parseResult
result=uint8(0);
if ~coder.target('SFun')
    coder.ceval('getResult',coder.ref(result));    
end

== matlab function RaspPiPilot/messageParser/While Iterator Subsystem/attitudeParser/MATLAB Function1 ==
  data: roll output; pitch output
function [roll,pitch] = parseRollPitch()
roll=double(0);
pitch=double(0);
if ~coder.target('SFun')
    coder.ceval('getRoll',coder.ref(roll));
    coder.ceval('getPitch',coder.ref(pitch));
end

== stateflow chart RaspPiPilot/Chart ==
  state mainLoop [parallel]
    settings: executionOrder=1
    state Initializing
      state EstablishingConnection
        en:hbCount=1;
        du:if idsReceived(1)==1 hbCount=hbCount+1; end
      state requestingAtitude
        du:if every(10,tick)
        [dataOut,lengthOut] = requestStreams(uint8(10));
        send(sendme);
        end
      note: use more states for other streams if neccessary#
          |  and have super transition out of the last one
      (default) -> EstablishingConnection
      EstablishingConnection -> requestingAtitude : [hbCount==5]
    note: wait for 5 heartBeats
    note: request streams one  by one,
        | if data  not received after
        | 1 sec- request again
    state Ground
      entry: [dataOut,lengthOut] = sendArmDisarmFun(0);
      send(sendme);
      during:
      if joystickInput.arm && every(25,tick)
      [dataOut,lengthOut] = sendArmDisarmFun(1);
      send(sendme);
      end
    state Sky
      du:
      if joystickInput.disarm==1&& every(5,tick)
      [dataOut,lengthOut] = sendArmDisarmFun(0);
      send(sendme);
      end
      state Manual
        during:
        if joystickInput.prtyUp
        [dataOut,lengthOut] =sendRPYT(joystickInput.prty(1),...
        joystickInput.prty(2),...
        joystickInput.prty(3),...
        joystickInput.prty(4) );
        send(sendme);
        end
      state Autonomous
        entry: navOn=1;
        exit: navOn=0;
      (default) -> Manual
      Manual -> Autonomous : [joystickInput.nav]
      Autonomous -> Manual : [~joystickInput.nav]
    (default) -> Initializing
    requestingAtitude -> Ground : [idsReceived(31)==1]
    Sky -> Ground : [armStatus==0]
    Ground -> Sky : [armStatus==1]
  state FailSaves [parallel]
    settings: executionOrder=2
  data: data function_output; length function_output; streamId function_input; data function_output; length function_output; armdisarm function_input; data function_output; length function_output; R function_input; P function_input; Y function_input; T function_input; dataOut output; lengthOut output; navOn output; armStatus input size=1; idsReceived input size=256; hbCount local; joystickInput input Bus: JoystickBus size=1
  events: sendme output FUNCTION_CALL_EVENT
  function [data,length] = requestStreams(streamId):
    | function  [data,length] = requestStreams(streamId)
    | data2 = zeros(256,1,'uint8');
    | length =uint8(0);
    | data=data2;
    | if ~coder.target('SFun')
    |   length=coder.ceval('requestStream', coder.ref(data2),uint8(streamId));
    | 
    |   
    |   data=data2;
    | end
  function [data,length] = sendArmDisarmFun(armdisarm):
    | function  [data,length] = sendArmDisarmFun(armdisarm)
    | data2 = zeros(256,1,'uint8');
    | length =uint8(0);
    | data=data2;
    | if ~coder.target('SFun')
    |   length=coder.ceval('sendArmDisarm', coder.ref(data2),uint8(armdisarm));
    |   data=data2;  
    | end
  function [data,length] = sendRPYT(R, P, Y, T):
    | function  [data,length] = sendRPYT(R, P, Y, T)
    | data2 = zeros(256,1,'uint8');
    | length =uint8(0);
    | data=data2;
    | if ~coder.target('SFun')
    |     length=coder.ceval('sendRPYT',...
    |         coder.ref(data2),uint16(R),uint16(P),uint16(Y),uint16(T));
    |     data=data2;
    | end

== matlab function RaspPiPilot/messageParser/While Iterator Subsystem/stringParser/MATLAB Function1 ==
function parseString
if ~coder.target('SFun')
    coder.ceval('getString');    
end

== matlab function RaspPiPilot/Navigation/Function-Call Subsystem/parseBlues/ParseLandmark/MATLAB Function ==
  data: inputCentroids input; centroids data_store_memory; itt input
function fcn(inputCentroids, itt)
global centroids;
centroids(:,:,itt)=inputCentroids;

== matlab function RaspPiPilot/SerialRead ==
  data: data output; length output; spHandle data_store_memory
function [data,length]=serialRead
global spHandle;
data = zeros(512,1,'uint8');
length =int32(0);
if ~coder.target('SFun')
    if spHandle>0
        bytesRead = int32(0);
        dataRead = zeros(512,1,'uint8');
        bytesRead = coder.ceval('read',spHandle, coder.ref(dataRead), uint32(512));
        if bytesRead>0
            data= dataRead;
            length=bytesRead;
        end
    end
end

== matlab function RaspPiPilot/Navigation/Function-Call Subsystem/findBlue/MATLAB Function1 ==
  data: R input; blueIntensity output; G input; B input
function blueIntensity  = fcn(R,G,B)
%#codegen

blueIntensity = B - R*2/3 - G*2/3;

== matlab function RaspPiPilot/SerialInitilization ==
  data: spHandle data_store_memory
function initSerial
global spHandle;
if ~coder.target('SFun')   
    if isempty(spHandle)||spHandle==-1;
        spHandle=int32(0);
        spHandle =coder.ceval('setupSerialPort',['/dev/ttyAMA0' 0], uint32(57600));
        
    end 
end

== matlab function RaspPiPilot/Navigation/Function-Call Subsystem/findBlue/MATLAB Function ==
  data: centroid_largest output; area input; centroid input; bbox_largest output; bbox input
function [centroid_largest, bbox_largest] = selectLargest(area, centroid, bbox)
[y, i] = sort(area);
l=length(area);
bbox_largest = [bbox(i(l),:); bbox(i(l-1),:) ;bbox(i(l-2),:);bbox(i(l-3),:) ];
centroid_largest = [centroid(i(l),:); centroid(i(l-1),:) ;centroid(i(l-2),:);centroid(i(l-3),:) ];

== matlab function RaspPiPilot/Navigation/MATLAB Function ==
  data: centroidMat output; centroids data_store_memory
function centroidMat = fcn
global centroids;
centroidMat=int16([centroids(:,:,1);centroids(:,:,2);centroids(:,:,3);centroids(:,:,4)]);

== matlab function RaspPiPilot/messageParser/While Iterator Subsystem/statusParser/MATLAB Function1 ==
function parseStatus
if ~coder.target('SFun')
    coder.ceval('parseSysStatus');    
end

== matlab function RaspPiPilot/messageParser/While Iterator Subsystem/heartBeatParser/MATLAB Function1 ==
  data: armed output
function armed =parseHeartbeat
status=uint8(0);
armed=uint8(0);
if ~coder.target('SFun')
    status=coder.ceval('parseHeartBeat'); 
  armed= bitget(status,8);
end

== matlab function RaspPiPilot/Navigation/Function-Call Subsystem/parseBlues/ParseLandmark/Detect Colors/MATLAB Function2 ==
  data: R input; RI output size=[320 240]; GI output size=[320  240]; YI output size=[320  240]; PI output size=[320  240]; G input; B input
function [RI, GI,YI,PI] = fcn(R,G,B)
RI = R - G - B;
GI = G - R - B;
YI = R + G - 3*B;
PI = R + B - 3*G;

== matlab function RaspPiPilot/Navigation/Function-Call Subsystem/parseBlues/ParseLandmark/MATLAB Function2 ==
  data: pos input; itt input; positionData data_store_memory
function writePos(pos, itt)
global positionData;
positionData(itt,:)=pos;

== matlab function RaspPiPilot/Navigation/Function-Call Subsystem/parseBlues/If Action Subsystem1/MATLAB Function1 ==
  data: itt input; positionData data_store_memory
function fcn( itt)
global positionData;
positionData(itt,:)=[-1000 -1000];

== matlab function RaspPiPilot/Navigation/MATLAB Function1 ==
  data: position output; positionData data_store_memory; positionAvailable output
function [position ,positionAvailable] = getPosition
global positionData;
positionAvailable=zeros(1,4);
position=[0 0];
for i=1:4
if positionData(i,1)~=-1000
    position=(position+positionData(i,:));
    positionAvailable(1,i)=1;
end
end
position=position/sum(positionAvailable,2);

== matlab function RaspPiPilot/Navigation/Function-Call Subsystem/parseBlues/ParseLandmark/MATLAB Function1 ==
  data: distance input; X output; heading input; rotation input; offset input; R output; y output
function [X, R,y] = fcn(distance,heading,rotation,offset)
X_local = -distance*[sin(rotation(1)); -sin(rotation(2))];
R = [cos(-heading) sin(-heading); -sin(-heading) cos(-heading)];
% X = [R*X_local+offset';distance;heading];
y=R*X_local;
X=[R*X_local+offset'];

== matlab function RaspPiPilot/Navigation/Function-Call Subsystem/parseBlues/ParseLandmark/attitudeFix/MATLAB Function ==
  data: pitch input; c output; roll input; angle input
function c = fcn(pitch,roll,angle)
alfa=sqrt((pitch-angle(1))^2 +(roll-angle(2))^2);
c=1/cos(alfa);
